simulink model "untitled11"  (R2018b)
settings: Solver=VariableStepAuto  StartTime=0.0  StopTime=10.0  RelTol=1e-3
libraries: fuzblock x1
settings Model: Creator=Tara  LastModifiedBy=Tara

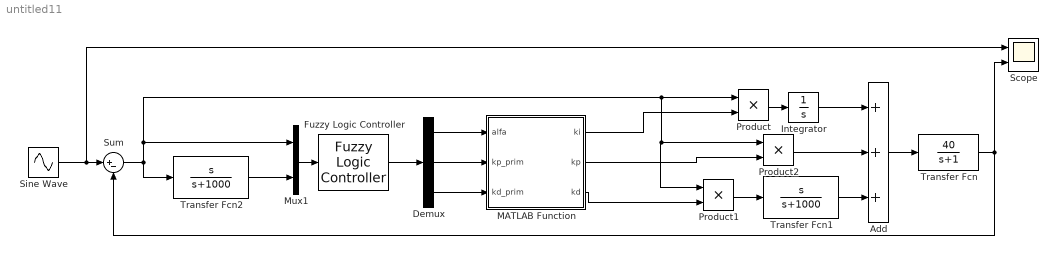
== system untitled11 ==
  Add : Sum  Inputs=+++
  Demux : Demux  Outputs=3
  Fuzzy Logic Controller : fuzblock/Fuzzy Logic  Controller  FIS='fuzzy.fis'  OutputSampleNumber=101  DataType=double  FuzzifiedInputs=off  RuleFiringStrengths=off  RuleOutputs=off  AggregatedOutputs=off  SimulateUsing=Interpreted execution  OutOfRangeInputValueMessage=warning  NoRuleFiredMessage=warning  EmptyOutputFuzzySetMessage=warning
  Integrator : Integrator
  MATLAB Function : MATLAB Function  TreatAsAtomicUnit=on
  Mux1 : Mux  Inputs=2
  Product : Product
  Product1 : Product
  Product2 : Product
  Scope : Scope  NumInputPorts=2
  Sine Wave : Sin  SampleTime=0
  Sum : Sum  Inputs=|+-
  Transfer Fcn : TransferFcn  Numerator=[40]  Denominator=[1 1]
  Transfer Fcn1 : TransferFcn  Numerator=[1,0]  Denominator=[1 1000]
  Transfer Fcn2 : TransferFcn  Numerator=[1,0]  Denominator=[1 1000]
  wires:
  Fuzzy Logic Controller/1 -> Demux/1
  Demux/1 -> MATLAB Function/1(alfa)
  Demux/2 -> MATLAB Function/2(kp_prim)
  Demux/3 -> MATLAB Function/3(kd_prim)
  Sine Wave/1 -> Scope/1, Sum/1
  Transfer Fcn/1 -> Sum/2, Scope/2
  Sum/1 -> Transfer Fcn2/1, Mux1/1, Product1/1, Product2/1, Product/1
  Mux1/1 -> Fuzzy Logic Controller/1
  Integrator/1 -> Add/1
  Transfer Fcn1/1 -> Add/3
  Add/1 -> Transfer Fcn/1
  MATLAB Function/1(ki) -> Product/2
  Product/1 -> Integrator/1
  Product2/1 -> Add/2
  MATLAB Function/2(kp) -> Product2/2
  Product1/1 -> Transfer Fcn1/1
  MATLAB Function/3(kd) -> Product1/2
  Transfer Fcn2/1 -> Mux1/2

== matlab function untitled11/MATLAB Function ==
  data: alfa input; ki output; kp_prim input; kd_prim input; kp output; kd output
function [ki,kp,kd] = fcn(alfa,kp_prim,kd_prim)
kp = 5*kp_prim;
kd = 5*kd_prim;
ki = (kp^2)/(alfa*kd);

% ki=kd/a;
